simulink model "CruiseControlSystem"  (Simulink 8.3)
settings: Solver=ode1  StartTime=0.0  StopTime=10.0  RelTol=1e-3
undefined symbols (not defined in the file): DiscIntNeverNeededParam
settings Model: Creator=gwilli10  LastModifiedBy=anthonydelage
settings DataIOCC: SignalLoggingSaveFormat=Dataset
settings OptimizationCC: OptimizeModelRefInitCode=on  LifeSpan=1
settings DebuggingCC: UnderspecifiedInitializationDetection=Simplified  StateNameClashWarn=none
settings HardwareCC: ProdIntDivRoundTo=Floor  ProdEndianess=LittleEndian  ProdHWDeviceType=Generic->32-bit Embedded Processor
settings RTWCC: SystemTargetFile=ert.tlc  GenCodeOnly=on  TemplateMakefile=ert_default_tmf  Description=Embedded Coder  ProcessScript=ert_make_rtw_hook
settings CodeAppCC: IgnoreCustomStorageClasses=off  MATLABSourceComments=on
settings ERTTargetCC: MultiwordLength=2048  GenerateSampleERTMain=on  ERTCustomFileTemplate=example_file_process.tlc  ERTFilePackagingFormat=CompactWithDataFile  SuppressUnreachableDefaultCases=off

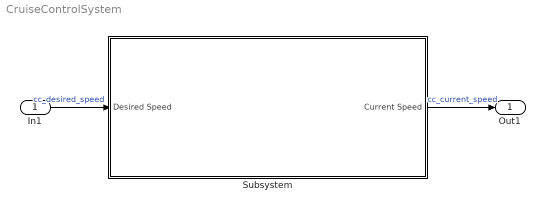
== system CruiseControlSystem ==
  In1 : Inport
  Subsystem : Subsystem
  Out1 : Outport
  wires:
  In1/1 -> Subsystem/1(Desired Speed)  "cc_desired_speed"
  Subsystem/1(Current Speed) -> Out1/1  "cc_current_speed"

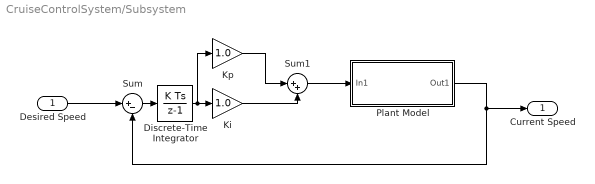
== system CruiseControlSystem/Subsystem ==
  Desired Speed : Inport
  Discrete-Time Integrator : DiscreteIntegrator  ICPrevOutput=DiscIntNeverNeededParam  ICPrevScaledInput=DiscIntNeverNeededParam
  Ki : Gain  Gain=1.0
  Kp : Gain  Gain=1.0
  "Plant Model " : Subsystem
  Sum : Sum  Inputs=|+-
  Sum1 : Sum  Inputs=|++
  Current Speed : Outport
  wires:
  "Plant Model "/1(Out1) -> Current Speed/1, Sum/2
  Discrete-Time Integrator/1 -> Kp/1, Ki/1
  Ki/1 -> Sum1/2
  Kp/1 -> Sum1/1
  Sum1/1 -> "Plant Model "/1(In1)
  Desired Speed/1 -> Sum/1
  Sum/1 -> Discrete-Time Integrator/1

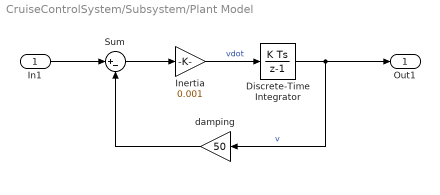
== system CruiseControlSystem/Subsystem/Plant Model  ==
  In1 : Inport
  Discrete-Time Integrator : DiscreteIntegrator  ICPrevOutput=DiscIntNeverNeededParam  ICPrevScaledInput=DiscIntNeverNeededParam
  "Inertia " : Gain  Gain=0.001
  Sum : Sum  Inputs=|+-
  damping : Gain  Gain=50
  Out1 : Outport
  wires:
  Discrete-Time Integrator/1 -> Out1/1, damping/1  "v"
  damping/1 -> Sum/2
  Sum/1 -> "Inertia "/1
  In1/1 -> Sum/1
  "Inertia "/1 -> Discrete-Time Integrator/1  "vdot"
